simulink model "Model_Guido_v4"  (R2021b)
settings: Solver=ode23tb  StartTime=0.0  StopTime=21  RelTol=1e-6
InitFcn:
  | Jrobot = ...
  | 9.06e-09 + 2.7656e-06 + 7.9365e-06
undefined symbols (not defined in the file): Bvx, Bvy, Bw, C, Cvx, Cvy, Cw, D, d, DiscIntNeverNeededParam, Gam, J, K_fsfb, K_int, Kt, l, M, Phi, r, Ti, Ts
libraries: slpidlib x3
settings Model: Creator=User  LastModifiedBy=user
settings SolverCC: ZeroCrossControl=EnableAll  ZeroCrossAlgorithm=Adaptive  AlgebraicLoopSolver=TrustRegion
settings DebuggingCC: IgnoredZcDiagnostic=none  SFMachineParentedDataDiag=warning

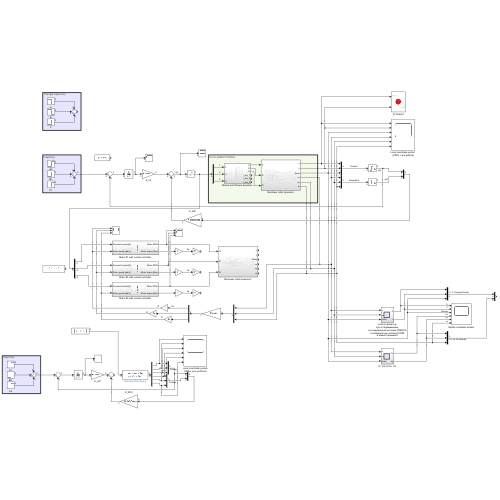
[thumbnail: Simulink's stored preview of the top-level diagram]
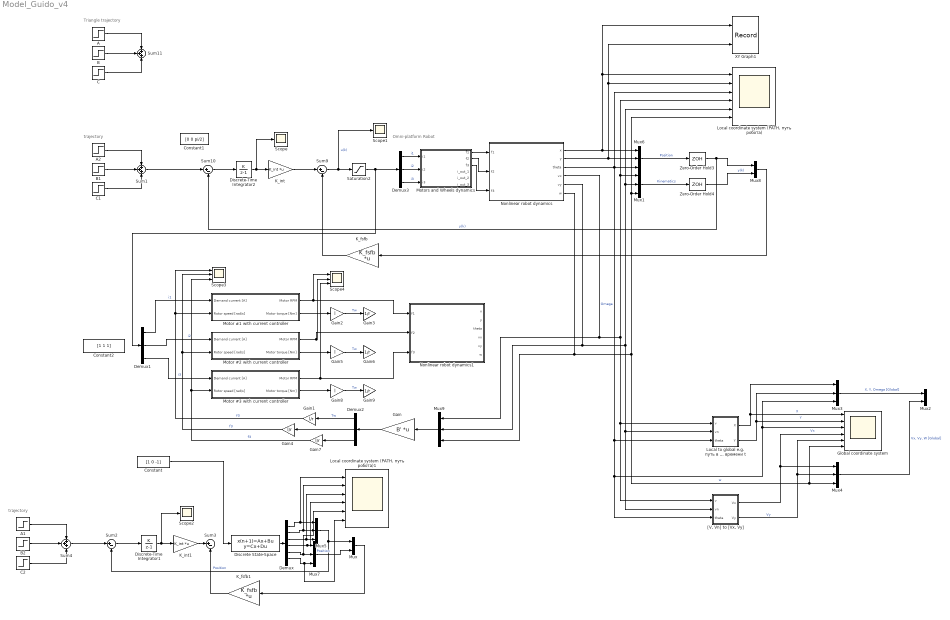
== system Model_Guido_v4 ==
  note: Omni-platform Robot
  note: Triangle trajectory
  note: trajectory
  note: trajectory
  A : Step  Time=0  Before=[1 0.5 pi/2]  After=[0.5 -sqrt(3)/2 1]  SampleTime=Ts
  A1 : Step  Time=0  Before=[0 0 0]  After=[1 1 0]  SampleTime=Ts
  A2 : Step  Time=0  Before=[0 0 0]  After=[1 1 0]  SampleTime=Ts
  B : Step  Time=6  Before=[0 0 0]  After=[-1 0 1]  SampleTime=Ts
  B1 : Step  Time=6  Before=[0 0 0]  After=[0 0 pi]  SampleTime=Ts
  B2 : Step  Time=6  Before=[0 0 0]  After=[0 0 pi]  SampleTime=Ts
  C : Step  Time=12  Before=[0 0 0]  After=[0.5 sqrt(3)/2 0]  SampleTime=Ts
  C1 : Step  Time=12  Before=[0 0 0]  After=[1 1 0]  SampleTime=Ts
  C2 : Step  Time=12  Before=[0 0 0]  After=[1 1 0]  SampleTime=Ts
  Constant : Constant  Value=[1 0 -1]  SampleTime=Ts
  Constant1 : Constant  Value=[0 0 pi/2]  SampleTime=Ts
  Constant2 : Constant  Value=[1 1 1]
  Demux : Demux  Outputs=6
  Demux1 : Demux  Outputs=3
  Demux2 : Demux  Outputs=3
  Demux3 : Demux  Outputs=3
  Discrete State-Space : DiscreteStateSpace  A=Phi  B=Gam  C=C  D=D  SampleTime=Ts
  Discrete-Time Integrator1 : DiscreteIntegrator  IntegratorMethod=Accumulation: Forward Euler  InitialCondition=[ 0 0 0]  SampleTime=Ts  ICPrevOutput=DiscIntNeverNeededParam  ICPrevScaledInput=DiscIntNeverNeededParam
  Discrete-Time Integrator2 : DiscreteIntegrator  IntegratorMethod=Accumulation: Forward Euler  InitialCondition=[ 0 0 0]  SampleTime=Ts  ICPrevOutput=DiscIntNeverNeededParam  ICPrevScaledInput=DiscIntNeverNeededParam
  Gain : Gain  Gain=B'  Multiplication=Matrix(K*u) (u vector)
  Gain1 : Gain  Gain=l/r
  Gain2 : Gain  Gain=l
  Gain3 : Gain  Gain=1/r
  Gain4 : Gain  Gain=l/r
  Gain5 : Gain  Gain=l
  Gain6 : Gain  Gain=1/r
  Gain7 : Gain  Gain=l/r
  Gain8 : Gain  Gain=l
  Gain9 : Gain  Gain=1/r
  Global coordinate system : Scope  NumInputPorts=6
  K_fsfb : Gain  Gain=K_fsfb  Multiplication=Matrix(K*u) (u vector)
  K_fsfb1 : Gain  Gain=K_fsfb  Multiplication=Matrix(K*u) (u vector)
  K_int : Gain  Gain=K_int  Multiplication=Matrix(K*u) (u vector)
  K_int1 : Gain  Gain=K_int  Multiplication=Matrix(K*u) (u vector)
  "Local coordinate system (PATH, путь робота)" : Scope  NumInputPorts=6
  "Local coordinate system (PATH, путь робота)1" : Scope  NumInputPorts=6
  "Local to global e.g. путь в перемещение, из координатной системы РОБОТА в координатную систему ПОЛЯ в момент времени t" : Subsystem
  Motor #1 with current controller : Subsystem
  Motor #2 with current controller : Subsystem
  Motor #3 with current controller : Subsystem
  "Motors and Wheels dynamics " : Subsystem
  Mux : Mux  Inputs=2
  Mux{1,3..7,9} (7 alike) : Mux  Inputs=3
  Mux2 : Mux  Inputs=2
  Mux8 : Mux  Inputs=2
  Nonlinear robot dynamics : Subsystem
  Nonlinear robot dynamics1 : Subsystem
  Saturation2 : Saturate  UpperLimit=3  LowerLimit=-3
  Scope : Scope
  Scope1 : Scope
  Scope2 : Scope
  Scope3 : Scope  NumInputPorts=3
  Scope4 : Scope  NumInputPorts=3
  Sum1 : Sum  Inputs=+++
  Sum{2..3,9..10} (4 alike) : Sum  Inputs=|+-
  Sum11 : Sum  Inputs=+++
  Sum4 : Sum  Inputs=+++
  XY Graph1 : Record  FileSettingsInternal="{\"entries\":[{\"content\":{\"excelSettings\":{\"content\":{},\"type\":\"Streamout.ExcelSettings\"}},\"type\":\"Streamout.FileSettingStorage\",\"uuid\":\"a91d3de9-fa65-4d7a-bf6d-cd6d2865a620\"}],\"packageUris\":[\"http://schema.mathworks.com/mf0/streamout_blocks/R2020a\"],\"version\":\"1.0\"}"  Layout=[1 1]  SignalsInternal="{\"entries\":[{\"content\":{\"signals\":[{\"content\":{\"blockPath\":[\"Model_Guido_v4/XY Graph1\"],\"channel\":[],\"dimensions\":[1],\"domain\":\"Model_Guido_v4/XY Graph1\",\"lineColor\":\"#64d413\",\"plots\":[],\"port\":1,\"sid\":[\"\"],\"signalID\":1754,\"signalName\":\"Nonlinear robot dynamics:1\"},\"type\":\"RecordBlkView.Signal\",\"uuid\":\"e1540467-9743-473a-afb9-9a18f09f25b7\"},{\"content\":{\"blockPath\":[\"Model_Guido_v4/XY Graph1\"],\"channel\":[],\"dimensions\":[1],\"domain\":\"Model_Guido_v4/XY Graph1\",\"lineColor\":\"#ff13a6\",\"plots\":[],\"port\":2,\"sid\":[\"\"],\"signalID\":1758,\"signalName\":\"Nonlinear robot dynamics:2\"},\"type\":\"RecordBlkView.Signal\",\"uuid\":\"eed5ca6f-00cb-43bc-9801-afdcc316eb87\"}]},\"type\":\"RecordBlkView.InputSignals\",\"uuid\":\"a4ae4625-cf57-4528-a4c5-005a48998e40\"}],\"packageUris\":[\"http://schema.mathworks.com/mf0/streamout_blocks/R2020a\"],\"version\":\"1.0\"}"  VisualizationBindings="{\"xyplotplugin\":{\"info\":[{\"series\":[],\"subplotID\":1}]}}"  CompatibilityTag=XY  st=-1
  Zero-Order Hold3 : ZeroOrderHold  SampleTime=Ts
  Zero-Order Hold4 : ZeroOrderHold  SampleTime=Ts
  "[V, Vn] to [Vx, Vy]" : Subsystem
  wires:
  Nonlinear robot dynamics/1(x) -> "Local coordinate system (PATH, путь робота)"/1, XY Graph1/1, Mux6/1
  Nonlinear robot dynamics/2(y) -> "Local coordinate system (PATH, путь робота)"/2, XY Graph1/2, Mux6/2
  Nonlinear robot dynamics/3(theta) -> "Local to global e.g. путь в перемещение, из координатной системы РОБОТА в координатную систему ПОЛЯ в момент времени t"/3(theta), "[V, Vn] to [Vx, Vy]"/3(theta), Mux3/3, Global coordinate system/3, "Local coordinate system (PATH, путь робота)"/3, Mux6/3  "Omega"
  Mux6/1 -> Zero-Order Hold3/1  "Position"
  C/1 -> Sum11/3
  Sum9/1 -> Scope1/1, Saturation2/1  "u(k)"
  Zero-Order Hold3/1 -> Mux8/1, Sum10/2  "y(k)"
  Discrete-Time Integrator2/1 -> Scope/1, K_int/1
  Sum10/1 -> Discrete-Time Integrator2/1
  A/1 -> Sum11/1
  B/1 -> Sum11/2
  Nonlinear robot dynamics/5(vy) -> Mux9/2, "Local to global e.g. путь в перемещение, из координатной системы РОБОТА в координатную систему ПОЛЯ в момент времени t"/2(vn), "[V, Vn] to [Vx, Vy]"/2(vn), Mux1/2, "Local coordinate system (PATH, путь робота)"/5
  Nonlinear robot dynamics/6(w) -> Mux9/3, Mux1/3, "Local coordinate system (PATH, путь робота)"/6, Global coordinate system/6, Mux4/3  "w"
  Nonlinear robot dynamics/4(vx) -> Mux9/1, "Local to global e.g. путь в перемещение, из координатной системы РОБОТА в координатную систему ПОЛЯ в момент времени t"/1(v), "[V, Vn] to [Vx, Vy]"/1(v), Mux1/1, "Local coordinate system (PATH, путь робота)"/4
  Demux3/1 -> "Motors and Wheels dynamics "/1(i1)  "i1"
  Demux3/2 -> "Motors and Wheels dynamics "/2(i2)  "i2"
  Demux3/3 -> "Motors and Wheels dynamics "/3(i3)  "i3"
  Zero-Order Hold4/1 -> Mux8/2  "y(k)"
  Mux1/1 -> Zero-Order Hold4/1  "Kinematics"
  Mux8/1 -> K_fsfb/1
  K_int/1 -> Sum9/1
  "Local to global e.g. путь в перемещение, из координатной системы РОБОТА в координатную систему ПОЛЯ в момент времени t"/1(X) -> Mux3/1, Global coordinate system/1  "X"
  "Local to global e.g. путь в перемещение, из координатной системы РОБОТА в координатную систему ПОЛЯ в момент времени t"/2(Y) -> Mux3/2, Global coordinate system/2  "Y"
  Mux3/1 -> Mux2/1  "X, Y, Omega [Global]"
  "[V, Vn] to [Vx, Vy]"/1(Vx) -> Global coordinate system/4, Mux4/1  "Vx"
  "[V, Vn] to [Vx, Vy]"/2(Vy) -> Global coordinate system/5, Mux4/2  "Vy"
  Mux4/1 -> Mux2/2  "Vx, Vy, W [Global]"
  C1/1 -> Sum1/3
  A2/1 -> Sum1/1
  B1/1 -> Sum1/2
  K_fsfb/1 -> Sum9/2
  K_int1/1 -> Sum3/1
  Sum2/1 -> Discrete-Time Integrator1/1
  Discrete-Time Integrator1/1 -> Scope2/1, K_int1/1
  Discrete State-Space/1 -> Demux/1
  C2/1 -> Sum4/3
  Sum4/1 -> Sum2/1
  A1/1 -> Sum4/1
  B2/1 -> Sum4/2
  Demux/1 -> "Local coordinate system (PATH, путь робота)1"/1, Mux5/1
  Demux/2 -> "Local coordinate system (PATH, путь робота)1"/2, Mux5/2
  Demux/3 -> "Local coordinate system (PATH, путь робота)1"/3, Mux5/3
  Demux/4 -> "Local coordinate system (PATH, путь робота)1"/4, Mux7/1
  Demux/5 -> "Local coordinate system (PATH, путь робота)1"/5, Mux7/2
  Demux/6 -> "Local coordinate system (PATH, путь робота)1"/6, Mux7/3
  Mux5/1 -> Mux/1, Sum2/2  "Position"
  K_fsfb1/1 -> Sum3/2
  Mux7/1 -> Mux/2  "Position"
  Mux/1 -> K_fsfb1/1
  Constant/1 -> Discrete State-Space/1
  Sum1/1 -> Sum10/1
  Gain5/1 -> Gain6/1  "Tw"
  Gain8/1 -> Gain9/1  "Tw"
  Gain2/1 -> Gain3/1  "Tw"
  Motor #1 with current controller/2(Motor torque [Nm]) -> Gain2/1
  Motor #2 with current controller/2(Motor torque [Nm]) -> Gain5/1
  Motor #3 with current controller/2(Motor torque [Nm]) -> Gain8/1
  Demux1/2 -> Motor #2 with current controller/1(Demand current [A])  "i2"
  Demux1/1 -> Motor #1 with current controller/1(Demand current [A])  "i1"
  Demux1/3 -> Motor #3 with current controller/1(Demand current [A])  "i3"
  Motor #1 with current controller/1(Motor RPM) -> Nonlinear robot dynamics1/1(f1), Scope4/1
  Motor #2 with current controller/1(Motor RPM) -> Nonlinear robot dynamics1/2(f2), Scope4/2
  Motor #3 with current controller/1(Motor RPM) -> Nonlinear robot dynamics1/3(f3), Scope4/3
  "Motors and Wheels dynamics "/1(f1) -> Nonlinear robot dynamics/1(f1)
  "Motors and Wheels dynamics "/2(f2) -> Nonlinear robot dynamics/2(f2)
  "Motors and Wheels dynamics "/3(f3) -> Nonlinear robot dynamics/3(f3)
  Saturation2/1 -> Demux1/1, Demux3/1
  Mux9/1 -> Gain/1
  Gain/1 -> Demux2/1
  Demux2/2 -> Gain4/1
  Demux2/3 -> Gain7/1
  Demux2/1 -> Gain1/1  "Tw"
  Gain1/1 -> Scope3/1, Motor #1 with current controller/2(Rotor speed [rad/s])  "f3"
  Gain4/1 -> Scope3/2, Motor #2 with current controller/2(Rotor speed [rad/s])  "f3"
  Gain7/1 -> Motor #3 with current controller/2(Rotor speed [rad/s]), Scope3/3  "f3"

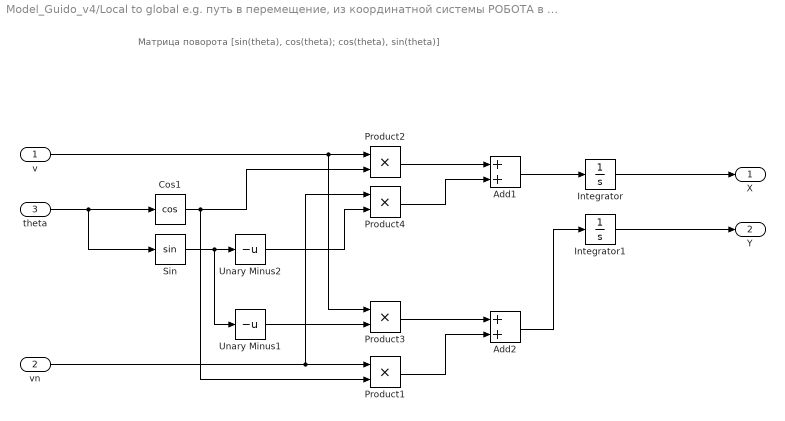
== system Model_Guido_v4/Local to global e.g. путь в перемещение, из координатной системы РОБОТА в координатную систему ПОЛЯ в момент времени t ==
  note: Матрица поворота
      | [sin(theta), cos(theta);
      |  cos(theta), sin(theta)]
  v : Inport
  vn : Inport  Port=2
  theta : Inport  Port=3
  Add1 : Sum
  Add2 : Sum
  Cos1 : Trigonometry  Operator=cos
  Integrator : Integrator
  Integrator1 : Integrator
  Product{1..4} (4 alike) : Product
  Sin : Trigonometry
  Unary Minus1 : UnaryMinus
  Unary Minus2 : UnaryMinus
  X : Outport
  Y : Outport  Port=2
  wires:
  Add1/1 -> Integrator/1
  Sin/1 -> Unary Minus1/1, Unary Minus2/1
  Product2/1 -> Add1/1
  Add2/1 -> Integrator1/1
  Product4/1 -> Add1/2
  Integrator1/1 -> Y/1
  v/1 -> Product3/1, Product2/1
  vn/1 -> Product4/1, Product1/1
  Product3/1 -> Add2/1
  Unary Minus1/1 -> Product3/2
  Product1/1 -> Add2/2
  Cos1/1 -> Product2/2, Product1/2
  theta/1 -> Sin/1, Cos1/1
  Integrator/1 -> X/1
  Unary Minus2/1 -> Product4/2

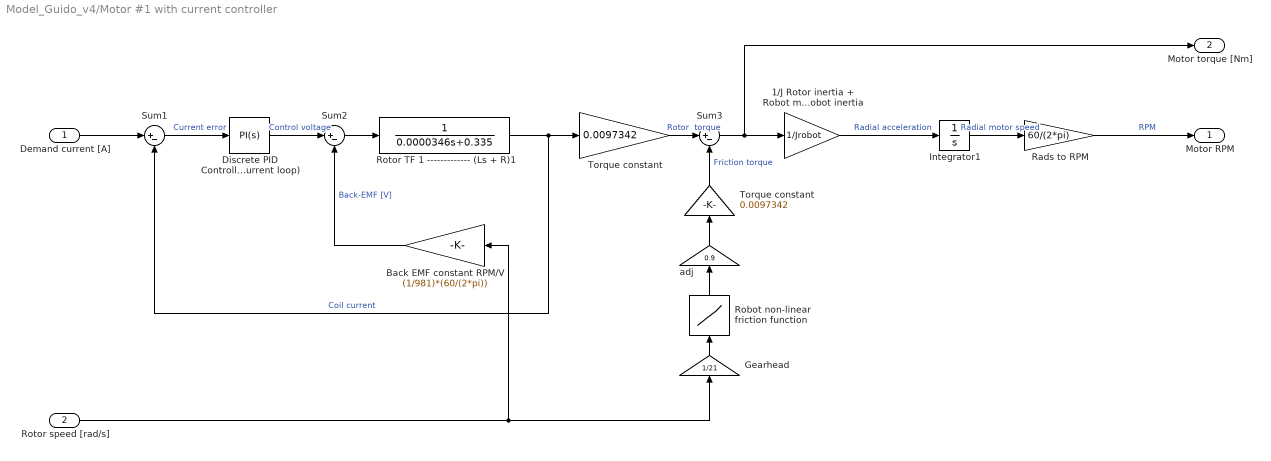
== system Model_Guido_v4/Motor #1 with current controller ==
  Demand current [A] : Inport
  Rotor speed [rad/s] : Inport  Port=2
  1/J Rotor inertia + Robot mass + Robot inertia : Gain  Gain=1/Jrobot
  Back EMF constant RPM/V : Gain  Gain=(1/981)*(60/(2*pi))
  Discrete PID Controller (current loop) : slpidlib/PID Controller  Controller=PI  Form=Parallel  TimeDomain=Continuous-time  UseExternalTs=off  SampleTime=1e-6  IntegratorMethod=Forward Euler  FilterMethod=Forward Euler  ControllerParametersSource=internal  P=291  I=291/(1e-6*237)  D=0  UseFilter=on  N=100  TunerSelectOption=Transfer Function Based (PID Tuner App)  InitialConditionSource=internal  InitialConditionForIntegrator=0  InitialConditionForFilter=0  DifferentiatorICPrevScaledInput=0  ExternalReset=none  TrackingMode=off  Kt=1  LimitOutput=on  SatLimitsSource=internal  UpperSaturationLimit=12  LowerSaturationLimit=-12  LinearizeAsGain=off  AntiWindupMode=none  Kb=1  POutMin=[]  POutMax=[]  IOutMin=[]  IOutMax=[]  DOutMin=[]  DOutMax=[]  NOutMin=[]  NOutMax=[]  SumOutMin=[]  SumOutMax=[]  SaturationOutMin=[]  SaturationOutMax=[]  PParamMin=[]  PParamMax=[]  IParamMin=[]  IParamMax=[]  DParamMin=[]  DParamMax=[]  NParamMin=[]  NParamMax=[]  KbParamMin=[]  KbParamMax=[]  KtParamMin=[]  KtParamMax=[]  KbOutMin=[]  KbOutMax=[]  KtOutMin=[]  KtOutMax=[]  IntegratorOutMin=[]  IntegratorOutMax=[]  FilterOutMin=[]  FilterOutMax=[]  SumI1OutMin=[]  SumI1OutMax=[]  SumI2OutMin=[]  SumI2OutMax=[]  SumI3OutMin=[]  SumI3OutMax=[]  SumI4OutMin=[]  SumI4OutMax=[]  SumDOutMin=[]  SumDOutMax=[]  DifferentiatorOutMin=[]  DifferentiatorOutMax=[]  FilterDiffOutCoefMin=[]  FilterDiffOutCoefMax=[]  ReciprocalOutMin=[]  ReciprocalOutMax=[]  SumDenOutMin=[]  SumDenOutMax=[]  SumNumOutMin=[]  SumNumOutMax=[]  DivideOutMin=[]  DivideOutMax=[]  UdiffTsProdOutMin=[]  UdiffTsProdOutMax=[]  NTsProdOutMin=[]  NTsProdOutMax=[]  UintegralTsProdOutMin=[]  UintegralTsProdOutMax=[]  UngainTsProdOutMin=[]  UngainTsProdOutMax=[]  IntegratorContinuousStateAttributes=''  IntegratorStateMustResolveToSignalObject=off  IntegratorRTWStateStorageClass=Auto  FilterContinuousStateAttributes=''  FilterStateMustResolveToSignalObject=off  FilterRTWStateStorageClass=Auto  ParallelPVariant=InternalParameters  IdealPVariant=Disabled  IVariant=InternalParameters  DVariant=Disabled  IntegratorVariant=Continuous  SatVariant=Enabled  AWVariant=Passthrough  PCopyVariant=Disabled  TRVariant=Disabled  FdbkBlocksVariant=Forward  IdealPFdbkVariant=Disabled  SatFdbkVariant=Disabled  DerivativeFilterVariant=Disabled  NVariant=Disabled  NCopyVariant=Disabled_SignalSpec  FilterICVariant=Disabled  IntegratorICVariant=InternalICs  ExternalResetVariant=Disabled  TRSumVariant=Passthrough  SumFdbkVariant=Disabled  SumVariant=Sum_PI  TsampFilterVariant=InternalTs  TsampNgainVariant=Passthrough  TsampIntegralVariant=Passthrough  ExternalSaturationOutDataTypeStr=Inherit: Same as second input
  "Gearhead " : Gain  Gain=1/21
  Integrator1 : Integrator
  Rads to RPM : Gain  Gain=60/(2*pi)
  Robot non-linear friction function : Lookup_n-D  NumberOfTableDimensions=1  BreakpointsForDimension1=[-38 -37 -0.01 0.01 37 38]  Table=[-2 -1.1 -0.5 0.5 1.1 2]  InternalRulePriority=Speed  RndMeth=Simplest  InputSameDT=on
  Rotor TF 1 ------------- (Ls + R)1 : TransferFcn  Denominator=[0.0000346 0.335]
  Sum1 : Sum  Inputs=|+-
  Sum2 : Sum  Inputs=|+-
  Sum3 : Sum  Inputs=|+-
  Torque constant : Gain  Gain=0.0097342
  "Torque constant " : Gain  Gain=0.0097342
  adj : Gain  Gain=0.9
  Motor RPM : Outport
  Motor torque [Nm] : Outport  Port=2
  wires:
  Discrete PID Controller (current loop)/1 -> Sum2/1  "Control voltage"
  Sum1/1 -> Discrete PID Controller (current loop)/1  "Current error"
  Rotor TF 1 ------------- (Ls + R)1/1 -> Torque constant/1, Sum1/2  "Coil current"
  Back EMF constant RPM/V/1 -> Sum2/2  "Back-EMF [V]"
  Sum2/1 -> Rotor TF 1 ------------- (Ls + R)1/1
  Torque constant/1 -> Sum3/1  "Rotor  torque"
  Robot non-linear friction function/1 -> adj/1
  Sum3/1 -> Motor torque [Nm]/1, 1/J Rotor inertia + Robot mass + Robot inertia/1
  "Gearhead "/1 -> Robot non-linear friction function/1
  Integrator1/1 -> Rads to RPM/1  "Radial motor speed"
  "Torque constant "/1 -> Sum3/2  "Friction torque"
  Demand current [A]/1 -> Sum1/1
  Rads to RPM/1 -> Motor RPM/1  "RPM"
  adj/1 -> "Torque constant "/1
  1/J Rotor inertia + Robot mass + Robot inertia/1 -> Integrator1/1  "Radial acceleration"
  Rotor speed [rad/s]/1 -> "Gearhead "/1, Back EMF constant RPM/V/1

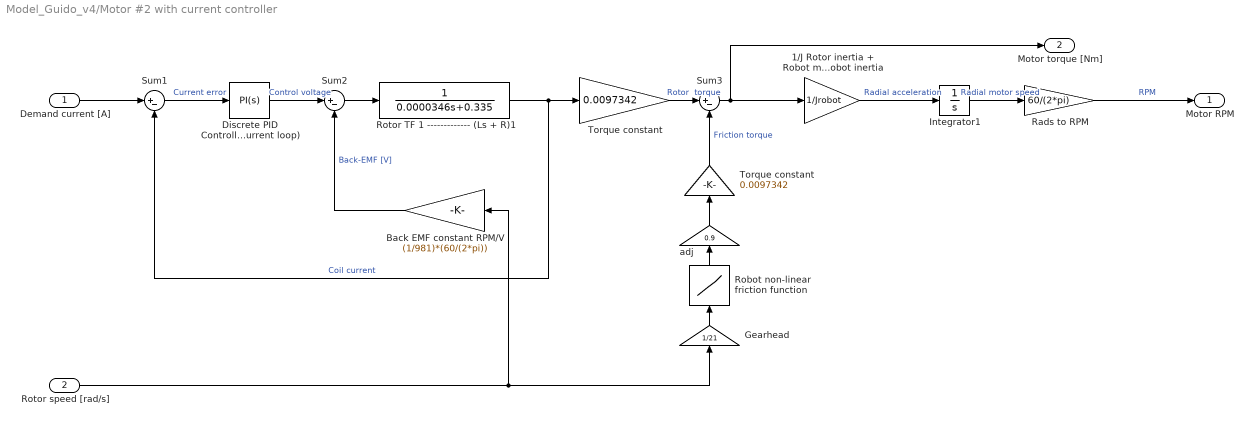
== system Model_Guido_v4/Motor #2 with current controller ==
  Demand current [A] : Inport
  Rotor speed [rad/s] : Inport  Port=2
  1/J Rotor inertia + Robot mass + Robot inertia : Gain  Gain=1/Jrobot
  Back EMF constant RPM/V : Gain  Gain=(1/981)*(60/(2*pi))
  Discrete PID Controller (current loop) : slpidlib/PID Controller  Controller=PI  Form=Parallel  TimeDomain=Continuous-time  UseExternalTs=off  SampleTime=1e-6  IntegratorMethod=Forward Euler  FilterMethod=Forward Euler  ControllerParametersSource=internal  P=291  I=291/(1e-6*237)  D=0  UseFilter=on  N=100  TunerSelectOption=Transfer Function Based (PID Tuner App)  InitialConditionSource=internal  InitialConditionForIntegrator=0  InitialConditionForFilter=0  DifferentiatorICPrevScaledInput=0  ExternalReset=none  TrackingMode=off  Kt=1  LimitOutput=on  SatLimitsSource=internal  UpperSaturationLimit=12  LowerSaturationLimit=-12  LinearizeAsGain=off  AntiWindupMode=none  Kb=1  POutMin=[]  POutMax=[]  IOutMin=[]  IOutMax=[]  DOutMin=[]  DOutMax=[]  NOutMin=[]  NOutMax=[]  SumOutMin=[]  SumOutMax=[]  SaturationOutMin=[]  SaturationOutMax=[]  PParamMin=[]  PParamMax=[]  IParamMin=[]  IParamMax=[]  DParamMin=[]  DParamMax=[]  NParamMin=[]  NParamMax=[]  KbParamMin=[]  KbParamMax=[]  KtParamMin=[]  KtParamMax=[]  KbOutMin=[]  KbOutMax=[]  KtOutMin=[]  KtOutMax=[]  IntegratorOutMin=[]  IntegratorOutMax=[]  FilterOutMin=[]  FilterOutMax=[]  SumI1OutMin=[]  SumI1OutMax=[]  SumI2OutMin=[]  SumI2OutMax=[]  SumI3OutMin=[]  SumI3OutMax=[]  SumI4OutMin=[]  SumI4OutMax=[]  SumDOutMin=[]  SumDOutMax=[]  DifferentiatorOutMin=[]  DifferentiatorOutMax=[]  FilterDiffOutCoefMin=[]  FilterDiffOutCoefMax=[]  ReciprocalOutMin=[]  ReciprocalOutMax=[]  SumDenOutMin=[]  SumDenOutMax=[]  SumNumOutMin=[]  SumNumOutMax=[]  DivideOutMin=[]  DivideOutMax=[]  UdiffTsProdOutMin=[]  UdiffTsProdOutMax=[]  NTsProdOutMin=[]  NTsProdOutMax=[]  UintegralTsProdOutMin=[]  UintegralTsProdOutMax=[]  UngainTsProdOutMin=[]  UngainTsProdOutMax=[]  IntegratorContinuousStateAttributes=''  IntegratorStateMustResolveToSignalObject=off  IntegratorRTWStateStorageClass=Auto  FilterContinuousStateAttributes=''  FilterStateMustResolveToSignalObject=off  FilterRTWStateStorageClass=Auto  ParallelPVariant=InternalParameters  IdealPVariant=Disabled  IVariant=InternalParameters  DVariant=Disabled  IntegratorVariant=Continuous  SatVariant=Enabled  AWVariant=Passthrough  PCopyVariant=Disabled  TRVariant=Disabled  FdbkBlocksVariant=Forward  IdealPFdbkVariant=Disabled  SatFdbkVariant=Disabled  DerivativeFilterVariant=Disabled  NVariant=Disabled  NCopyVariant=Disabled_SignalSpec  FilterICVariant=Disabled  IntegratorICVariant=InternalICs  ExternalResetVariant=Disabled  TRSumVariant=Passthrough  SumFdbkVariant=Disabled  SumVariant=Sum_PI  TsampFilterVariant=InternalTs  TsampNgainVariant=Passthrough  TsampIntegralVariant=Passthrough  ExternalSaturationOutDataTypeStr=Inherit: Same as second input
  "Gearhead " : Gain  Gain=1/21
  Integrator1 : Integrator
  Rads to RPM : Gain  Gain=60/(2*pi)
  Robot non-linear friction function : Lookup_n-D  NumberOfTableDimensions=1  BreakpointsForDimension1=[-38 -37 -0.01 0.01 37 38]  Table=[-2 -1.1 -0.5 0.5 1.1 2]  InternalRulePriority=Speed  RndMeth=Simplest  InputSameDT=on
  Rotor TF 1 ------------- (Ls + R)1 : TransferFcn  Denominator=[0.0000346 0.335]
  Sum1 : Sum  Inputs=|+-
  Sum2 : Sum  Inputs=|+-
  Sum3 : Sum  Inputs=|+-
  Torque constant : Gain  Gain=0.0097342
  "Torque constant " : Gain  Gain=0.0097342
  adj : Gain  Gain=0.9
  Motor RPM : Outport
  Motor torque [Nm] : Outport  Port=2
  wires:
  Rads to RPM/1 -> Motor RPM/1  "RPM"
  Demand current [A]/1 -> Sum1/1
  "Torque constant "/1 -> Sum3/2  "Friction torque"
  Integrator1/1 -> Rads to RPM/1  "Radial motor speed"
  1/J Rotor inertia + Robot mass + Robot inertia/1 -> Integrator1/1  "Radial acceleration"
  "Gearhead "/1 -> Robot non-linear friction function/1
  Sum3/1 -> 1/J Rotor inertia + Robot mass + Robot inertia/1, Motor torque [Nm]/1
  Robot non-linear friction function/1 -> adj/1
  Torque constant/1 -> Sum3/1  "Rotor  torque"
  Sum2/1 -> Rotor TF 1 ------------- (Ls + R)1/1
  Back EMF constant RPM/V/1 -> Sum2/2  "Back-EMF [V]"
  Rotor TF 1 ------------- (Ls + R)1/1 -> Sum1/2, Torque constant/1  "Coil current"
  Sum1/1 -> Discrete PID Controller (current loop)/1  "Current error"
  Discrete PID Controller (current loop)/1 -> Sum2/1  "Control voltage"
  adj/1 -> "Torque constant "/1
  Rotor speed [rad/s]/1 -> Back EMF constant RPM/V/1, "Gearhead "/1

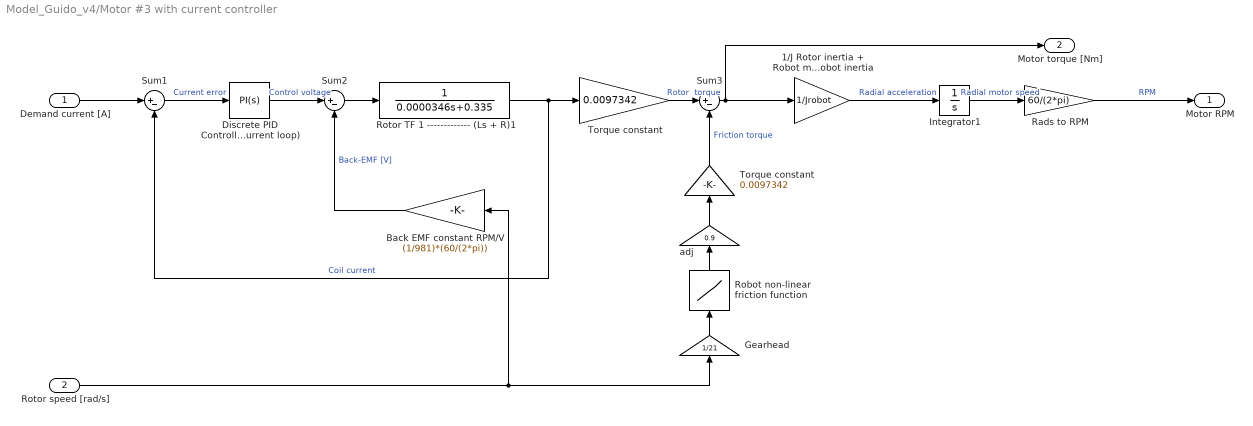
== system Model_Guido_v4/Motor #3 with current controller ==
  Demand current [A] : Inport
  Rotor speed [rad/s] : Inport  Port=2
  1/J Rotor inertia + Robot mass + Robot inertia : Gain  Gain=1/Jrobot
  Back EMF constant RPM/V : Gain  Gain=(1/981)*(60/(2*pi))
  Discrete PID Controller (current loop) : slpidlib/PID Controller  Controller=PI  Form=Parallel  TimeDomain=Continuous-time  UseExternalTs=off  SampleTime=1e-6  IntegratorMethod=Forward Euler  FilterMethod=Forward Euler  ControllerParametersSource=internal  P=291  I=291/(1e-6*237)  D=0  UseFilter=on  N=100  TunerSelectOption=Transfer Function Based (PID Tuner App)  InitialConditionSource=internal  InitialConditionForIntegrator=0  InitialConditionForFilter=0  DifferentiatorICPrevScaledInput=0  ExternalReset=none  TrackingMode=off  Kt=1  LimitOutput=on  SatLimitsSource=internal  UpperSaturationLimit=12  LowerSaturationLimit=-12  LinearizeAsGain=off  AntiWindupMode=none  Kb=1  POutMin=[]  POutMax=[]  IOutMin=[]  IOutMax=[]  DOutMin=[]  DOutMax=[]  NOutMin=[]  NOutMax=[]  SumOutMin=[]  SumOutMax=[]  SaturationOutMin=[]  SaturationOutMax=[]  PParamMin=[]  PParamMax=[]  IParamMin=[]  IParamMax=[]  DParamMin=[]  DParamMax=[]  NParamMin=[]  NParamMax=[]  KbParamMin=[]  KbParamMax=[]  KtParamMin=[]  KtParamMax=[]  KbOutMin=[]  KbOutMax=[]  KtOutMin=[]  KtOutMax=[]  IntegratorOutMin=[]  IntegratorOutMax=[]  FilterOutMin=[]  FilterOutMax=[]  SumI1OutMin=[]  SumI1OutMax=[]  SumI2OutMin=[]  SumI2OutMax=[]  SumI3OutMin=[]  SumI3OutMax=[]  SumI4OutMin=[]  SumI4OutMax=[]  SumDOutMin=[]  SumDOutMax=[]  DifferentiatorOutMin=[]  DifferentiatorOutMax=[]  FilterDiffOutCoefMin=[]  FilterDiffOutCoefMax=[]  ReciprocalOutMin=[]  ReciprocalOutMax=[]  SumDenOutMin=[]  SumDenOutMax=[]  SumNumOutMin=[]  SumNumOutMax=[]  DivideOutMin=[]  DivideOutMax=[]  UdiffTsProdOutMin=[]  UdiffTsProdOutMax=[]  NTsProdOutMin=[]  NTsProdOutMax=[]  UintegralTsProdOutMin=[]  UintegralTsProdOutMax=[]  UngainTsProdOutMin=[]  UngainTsProdOutMax=[]  IntegratorContinuousStateAttributes=''  IntegratorStateMustResolveToSignalObject=off  IntegratorRTWStateStorageClass=Auto  FilterContinuousStateAttributes=''  FilterStateMustResolveToSignalObject=off  FilterRTWStateStorageClass=Auto  ParallelPVariant=InternalParameters  IdealPVariant=Disabled  IVariant=InternalParameters  DVariant=Disabled  IntegratorVariant=Continuous  SatVariant=Enabled  AWVariant=Passthrough  PCopyVariant=Disabled  TRVariant=Disabled  FdbkBlocksVariant=Forward  IdealPFdbkVariant=Disabled  SatFdbkVariant=Disabled  DerivativeFilterVariant=Disabled  NVariant=Disabled  NCopyVariant=Disabled_SignalSpec  FilterICVariant=Disabled  IntegratorICVariant=InternalICs  ExternalResetVariant=Disabled  TRSumVariant=Passthrough  SumFdbkVariant=Disabled  SumVariant=Sum_PI  TsampFilterVariant=InternalTs  TsampNgainVariant=Passthrough  TsampIntegralVariant=Passthrough  ExternalSaturationOutDataTypeStr=Inherit: Same as second input
  "Gearhead " : Gain  Gain=1/21
  Integrator1 : Integrator
  Rads to RPM : Gain  Gain=60/(2*pi)
  Robot non-linear friction function : Lookup_n-D  NumberOfTableDimensions=1  BreakpointsForDimension1=[-38 -37 -0.01 0.01 37 38]  Table=[-2 -1.2 -0.55 0.55 1.2 2]  InternalRulePriority=Speed  RndMeth=Simplest  InputSameDT=on
  Rotor TF 1 ------------- (Ls + R)1 : TransferFcn  Denominator=[0.0000346 0.335]
  Sum1 : Sum  Inputs=|+-
  Sum2 : Sum  Inputs=|+-
  Sum3 : Sum  Inputs=|+-
  Torque constant : Gain  Gain=0.0097342
  "Torque constant " : Gain  Gain=0.0097342
  adj : Gain  Gain=0.9
  Motor RPM : Outport
  Motor torque [Nm] : Outport  Port=2
  wires:
  Discrete PID Controller (current loop)/1 -> Sum2/1  "Control voltage"
  Sum1/1 -> Discrete PID Controller (current loop)/1  "Current error"
  Rotor TF 1 ------------- (Ls + R)1/1 -> Torque constant/1, Sum1/2  "Coil current"
  Back EMF constant RPM/V/1 -> Sum2/2  "Back-EMF [V]"
  Sum2/1 -> Rotor TF 1 ------------- (Ls + R)1/1
  Torque constant/1 -> Sum3/1  "Rotor  torque"
  Robot non-linear friction function/1 -> adj/1
  Sum3/1 -> 1/J Rotor inertia + Robot mass + Robot inertia/1, Motor torque [Nm]/1
  1/J Rotor inertia + Robot mass + Robot inertia/1 -> Integrator1/1  "Radial acceleration"
  Integrator1/1 -> Rads to RPM/1  "Radial motor speed"
  "Torque constant "/1 -> Sum3/2  "Friction torque"
  Demand current [A]/1 -> Sum1/1
  Rads to RPM/1 -> Motor RPM/1  "RPM"
  "Gearhead "/1 -> Robot non-linear friction function/1
  adj/1 -> "Torque constant "/1
  Rotor speed [rad/s]/1 -> "Gearhead "/1, Back EMF constant RPM/V/1

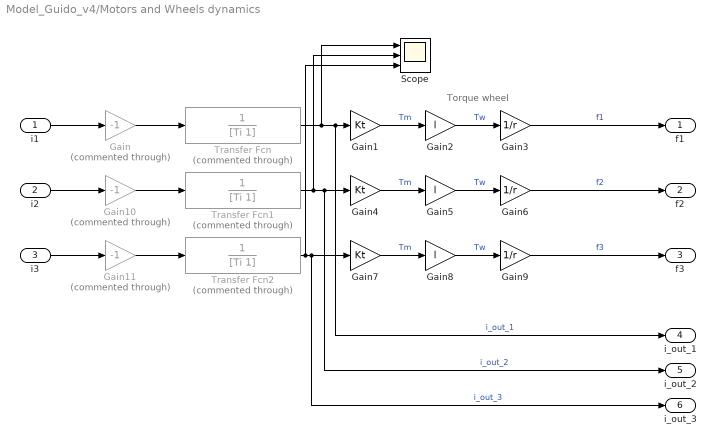
== system Model_Guido_v4/Motors and Wheels dynamics  ==
  note: Torque wheel
  i1 : Inport
  i2 : Inport  Port=2
  i3 : Inport  Port=3
  Gain : Gain  Commented=through  Gain=-1
  Gain1 : Gain  Gain=Kt
  Gain10 : Gain  Commented=through  Gain=-1
  Gain11 : Gain  Commented=through  Gain=-1
  Gain2 : Gain  Gain=l
  Gain3 : Gain  Gain=1/r
  Gain4 : Gain  Gain=Kt
  Gain5 : Gain  Gain=l
  Gain6 : Gain  Gain=1/r
  Gain7 : Gain  Gain=Kt
  Gain8 : Gain  Gain=l
  Gain9 : Gain  Gain=1/r
  Scope : Scope  NumInputPorts=3
  Transfer Fcn : TransferFcn  Commented=through  Denominator=[Ti 1]
  Transfer Fcn1 : TransferFcn  Commented=through  Denominator=[Ti 1]
  Transfer Fcn2 : TransferFcn  Commented=through  Denominator=[Ti 1]
  f1 : Outport
  f2 : Outport  Port=2
  f3 : Outport  Port=3
  i_out_1 : Outport  Port=4
  i_out_2 : Outport  Port=5
  i_out_3 : Outport  Port=6
  wires:
  i2/1 -> Gain10/1
  Gain1/1 -> Gain2/1  "Tm"
  Gain8/1 -> Gain9/1  "Tw"
  Gain5/1 -> Gain6/1  "Tw"
  Transfer Fcn/1 -> Scope/1, i_out_1/1, Gain1/1  "i_out_1"
  Transfer Fcn2/1 -> Scope/3, i_out_3/1, Gain7/1  "i_out_3"
  i3/1 -> Gain11/1
  Gain2/1 -> Gain3/1  "Tw"
  Gain7/1 -> Gain8/1  "Tm"
  Transfer Fcn1/1 -> Scope/2, i_out_2/1, Gain4/1  "i_out_2"
  Gain4/1 -> Gain5/1  "Tm"
  Gain3/1 -> f1/1  "f1"
  Gain6/1 -> f2/1  "f2"
  i1/1 -> Gain/1
  Gain9/1 -> f3/1  "f3"
  Gain/1 -> Transfer Fcn/1
  Gain10/1 -> Transfer Fcn1/1
  Gain11/1 -> Transfer Fcn2/1

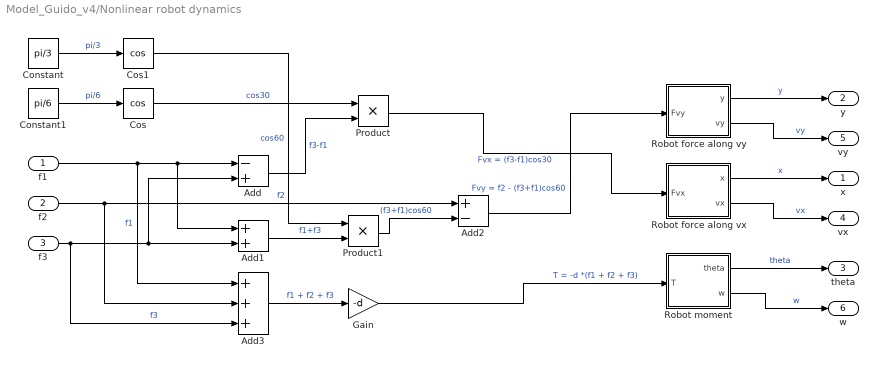
== system Model_Guido_v4/Nonlinear robot dynamics ==
  f1 : Inport
  f2 : Inport  Port=2
  f3 : Inport  Port=3
  Add : Sum  Inputs=-+
  Add1 : Sum
  Add2 : Sum  Inputs=+-
  Add3 : Sum  Inputs=+++
  Constant : Constant  Value=pi/3
  Constant1 : Constant  Value=pi/6
  Cos : Trigonometry  Operator=cos
  Cos1 : Trigonometry  Operator=cos
  Gain : Gain  Gain=-d
  Product : Product
  Product1 : Product
  Robot force along vx : Subsystem
  Robot force along vy : Subsystem
  Robot moment : Subsystem
  x : Outport
  y : Outport  Port=2
  theta : Outport  Port=3
  vx : Outport  Port=4
  vy : Outport  Port=5
  w : Outport  Port=6
  wires:
  f3/1 -> Add3/3, Add1/2, Add/2  "f3"
  f1/1 -> Add3/1, Add/1, Add1/1  "f1"
  f2/1 -> Add3/2, Add2/1  "f2"
  Robot force along vy/1(y) -> y/1  "y"
  Robot moment/1(theta) -> theta/1  "theta"
  Robot force along vx/2(vx) -> vx/1  "vx"
  Robot force along vx/1(x) -> x/1  "x"
  Robot moment/2(w) -> w/1  "w"
  Robot force along vy/2(vy) -> vy/1  "vy"
  Add/1 -> Product/2  "f3-f1"
  Constant1/1 -> Cos/1  "pi/6"
  Cos/1 -> Product/1  "cos30"
  Product/1 -> Robot force along vx/1(Fvx)  "Fvx = (f3-f1)cos30"
  Constant/1 -> Cos1/1  "pi/3"
  Cos1/1 -> Product1/1  "cos60"
  Add1/1 -> Product1/2  "f1+f3"
  Product1/1 -> Add2/2  "(f3+f1)cos60"
  Add2/1 -> Robot force along vy/1(Fvy)  "Fvy = f2 - (f3+f1)cos60"
  Add3/1 -> Gain/1  "f1 + f2 + f3"
  Gain/1 -> Robot moment/1(T)  "T = -d *(f1 + f2 + f3)"

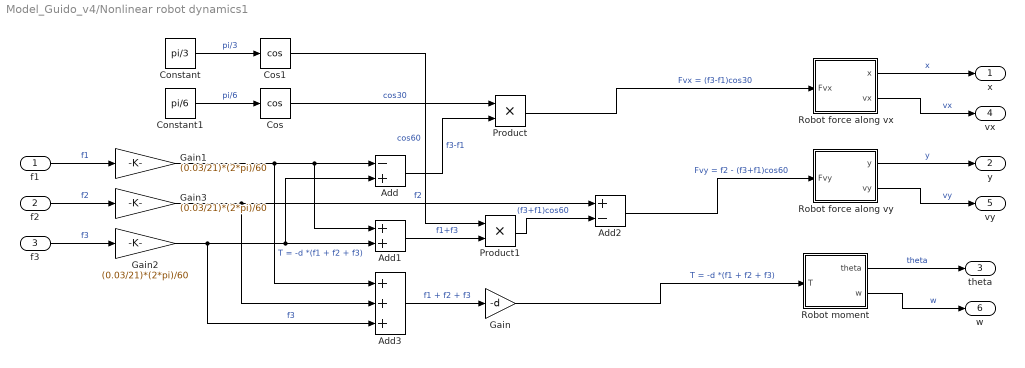
== system Model_Guido_v4/Nonlinear robot dynamics1 ==
  f1 : Inport
  f2 : Inport  Port=2
  f3 : Inport  Port=3
  Add : Sum  Inputs=-+
  Add1 : Sum
  Add2 : Sum  Inputs=+-
  Add3 : Sum  Inputs=+++
  Constant : Constant  Value=pi/3
  Constant1 : Constant  Value=pi/6
  Cos : Trigonometry  Operator=cos
  Cos1 : Trigonometry  Operator=cos
  Gain : Gain  Gain=-d
  Gain1 : Gain  Gain=(0.03/21)*(2*pi)/60
  Gain2 : Gain  Gain=(0.03/21)*(2*pi)/60
  Gain3 : Gain  Gain=(0.03/21)*(2*pi)/60
  Product : Product
  Product1 : Product
  Robot force along vx : Subsystem
  Robot force along vy : Subsystem
  Robot moment : Subsystem
  x : Outport
  y : Outport  Port=2
  theta : Outport  Port=3
  vx : Outport  Port=4
  vy : Outport  Port=5
  w : Outport  Port=6
  wires:
  Gain2/1 -> Add3/3, Add1/2, Add/2  "f3"
  f1/1 -> Gain1/1  "f1"
  Gain3/1 -> Add3/2, Add2/1  "f2"
  Robot force along vy/1(y) -> y/1  "y"
  Robot moment/1(theta) -> theta/1  "theta"
  Robot force along vx/2(vx) -> vx/1  "vx"
  Robot force along vx/1(x) -> x/1  "x"
  Robot moment/2(w) -> w/1  "w"
  Robot force along vy/2(vy) -> vy/1  "vy"
  Add/1 -> Product/2  "f3-f1"
  Constant1/1 -> Cos/1  "pi/6"
  Cos/1 -> Product/1  "cos30"
  Product/1 -> Robot force along vx/1(Fvx)  "Fvx = (f3-f1)cos30"
  Constant/1 -> Cos1/1  "pi/3"
  Cos1/1 -> Product1/1  "cos60"
  Add1/1 -> Product1/2  "f1+f3"
  Product1/1 -> Add2/2  "(f3+f1)cos60"
  Add2/1 -> Robot force along vy/1(Fvy)  "Fvy = f2 - (f3+f1)cos60"
  Add3/1 -> Gain/1  "f1 + f2 + f3"
  Gain/1 -> Robot moment/1(T)  "T = -d *(f1 + f2 + f3)"
  Gain1/1 -> Add3/1, Add/1, Add1/1  "T = -d *(f1 + f2 + f3)"
  f2/1 -> Gain3/1  "f2"
  f3/1 -> Gain2/1  "f3"

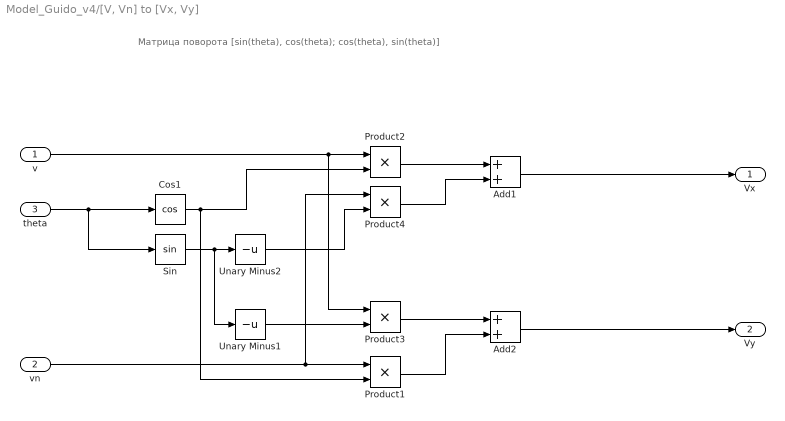
== system Model_Guido_v4/[V, Vn] to [Vx, Vy] ==
  note: Матрица поворота
      | [sin(theta), cos(theta);
      |  cos(theta), sin(theta)]
  v : Inport
  vn : Inport  Port=2
  theta : Inport  Port=3
  Add1 : Sum
  Add2 : Sum
  Cos1 : Trigonometry  Operator=cos
  Product{1..4} (4 alike) : Product
  Sin : Trigonometry
  Unary Minus1 : UnaryMinus
  Unary Minus2 : UnaryMinus
  Vx : Outport
  Vy : Outport  Port=2
  wires:
  Unary Minus2/1 -> Product4/2
  Add1/1 -> Vx/1
  theta/1 -> Cos1/1, Sin/1
  Cos1/1 -> Product1/2, Product2/2
  Product1/1 -> Add2/2
  Unary Minus1/1 -> Product3/2
  Product3/1 -> Add2/1
  vn/1 -> Product1/1, Product4/1
  v/1 -> Product2/1, Product3/1
  Add2/1 -> Vy/1
  Product4/1 -> Add1/2
  Product2/1 -> Add1/1
  Sin/1 -> Unary Minus2/1, Unary Minus1/1

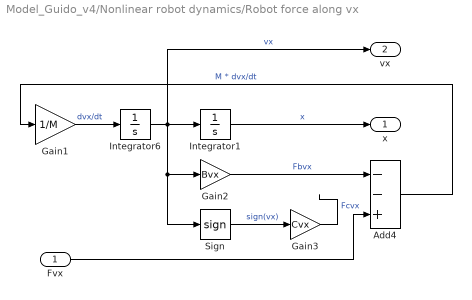
== system Model_Guido_v4/Nonlinear robot dynamics/Robot force along vx ==
  Fvx : Inport
  Add4 : Sum  Inputs=--+
  Gain1 : Gain  Gain=1/M
  Gain2 : Gain  Gain=Bvx
  Gain3 : Gain  Gain=Cvx
  Integrator1 : Integrator  ContinuousStateAttributes='x'
  Integrator6 : Integrator  ContinuousStateAttributes='vx'
  Sign : Signum
  x : Outport
  vx : Outport  Port=2
  wires:
  Fvx/1 -> Add4/3
  Sign/1 -> Gain3/1  "sign(vx)"
  Gain2/1 -> Add4/1  "Fbvx"
  Integrator1/1 -> x/1  "x"
  Integrator6/1 -> vx/1, Integrator1/1, Sign/1, Gain2/1  "vx"
  Gain1/1 -> Integrator6/1  "dvx/dt"
  Add4/1 -> Gain1/1  "M * dvx/dt"
  Gain3/1 -> ?  "Fcvx"

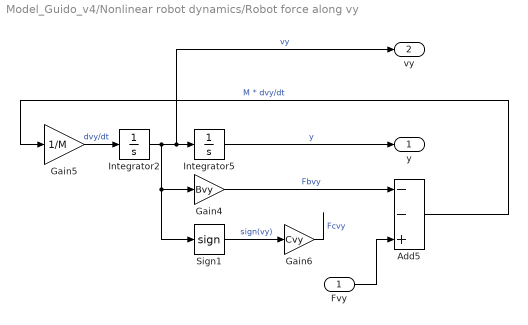
== system Model_Guido_v4/Nonlinear robot dynamics/Robot force along vy ==
  Fvy : Inport
  Add5 : Sum  Inputs=--+
  Gain4 : Gain  Gain=Bvy
  Gain5 : Gain  Gain=1/M
  Gain6 : Gain  Gain=Cvy
  Integrator2 : Integrator  ContinuousStateAttributes='vy'
  Integrator5 : Integrator  ContinuousStateAttributes='y'
  Sign1 : Signum
  y : Outport
  vy : Outport  Port=2
  wires:
  Gain5/1 -> Integrator2/1  "dvy/dt"
  Integrator2/1 -> vy/1, Integrator5/1, Sign1/1, Gain4/1  "vy"
  Fvy/1 -> Add5/3
  Add5/1 -> Gain5/1  "M * dvy/dt"
  Sign1/1 -> Gain6/1  "sign(vy)"
  Gain4/1 -> Add5/1  "Fbvy"
  Integrator5/1 -> y/1  "y"
  Gain6/1 -> ?  "Fcvy"

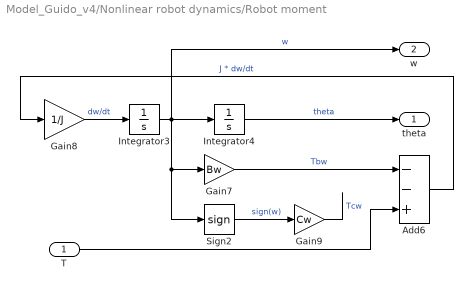
== system Model_Guido_v4/Nonlinear robot dynamics/Robot moment ==
  T : Inport
  Add6 : Sum  Inputs=--+
  Gain7 : Gain  Gain=Bw
  Gain8 : Gain  Gain=1/J
  Gain9 : Gain  Gain=Cw
  Integrator3 : Integrator  ContinuousStateAttributes='w'
  Integrator4 : Integrator  ContinuousStateAttributes='theta'
  Sign2 : Signum
  theta : Outport
  w : Outport  Port=2
  wires:
  Integrator3/1 -> w/1, Integrator4/1, Sign2/1, Gain7/1  "w"
  Gain8/1 -> Integrator3/1  "dw/dt"
  Add6/1 -> Gain8/1  "J * dw/dt"
  Gain7/1 -> Add6/1  "Tbw"
  Sign2/1 -> Gain9/1  "sign(w)"
  Integrator4/1 -> theta/1  "theta"
  T/1 -> Add6/3
  Gain9/1 -> ?  "Tcw"

== system Model_Guido_v4/Nonlinear robot dynamics1/Robot force along vx ==
  Fvx : Inport
  Integrator1 : Integrator  ContinuousStateAttributes='x'
  x : Outport
  vx : Outport  Port=2
  wires:
  Integrator1/1 -> x/1  "x"
  Fvx/1 -> vx/1, Integrator1/1  "vx"

== system Model_Guido_v4/Nonlinear robot dynamics1/Robot force along vy ==
  Fvy : Inport
  Integrator5 : Integrator  ContinuousStateAttributes='y'
  y : Outport
  vy : Outport  Port=2
  wires:
  Fvy/1 -> vy/1, Integrator5/1  "vy"
  Integrator5/1 -> y/1  "y"

== system Model_Guido_v4/Nonlinear robot dynamics1/Robot moment ==
  T : Inport
  Integrator4 : Integrator  ContinuousStateAttributes='theta'
  theta : Outport
  w : Outport  Port=2
  wires:
  T/1 -> w/1, Integrator4/1  "w"
  Integrator4/1 -> theta/1  "theta"
